simulink model "CM670A_HwAg1Meas"  (R2013b)
settings: Solver=FixedStepDiscrete  SolverMode=SingleTasking  StartTime=0.0  StopTime=22  FixedStep=0.002  RelTol=1e-3
values from neighbouring files (symbols this model uses):
  ELECGLBPRM_DEGPERREV_DEGPERREV_F32 = DataDict.Constant    [CM670A_HwAg1Meas_DataDict.m]
  ELECGLBPRM_HWAGCENTROFFS_HWDEG_F32 = DataDict.Constant    [CM670A_HwAg1Meas_DataDict.m]
  ELECGLBPRM_HWAGSATNLOWRLIM_HWDEG_F32 = DataDict.Constant    [CM670A_HwAg1Meas_DataDict.m]
  ELECGLBPRM_HWAGSATNUPPRLIM_HWDEG_F32 = DataDict.Constant    [CM670A_HwAg1Meas_DataDict.m]
  ELECGLBPRM_HWAGSCA_ULS_F32 = DataDict.Constant    [CM670A_HwAg1Meas_DataDict.m]
  ELECGLBPRM_HWAGSPURGEARRAT_ULS_F32 = DataDict.Constant    [CM670A_HwAg1Meas_DataDict.m]
  ELECGLBPRM_HWAGSPURTORINGGEARRATSNSR0_ULS_F32 = DataDict.Constant    [CM670A_HwAg1Meas_DataDict.m]
  ELECGLBPRM_HWAGSPURTORINGGEARRATSNSR1_ULS_F32 = DataDict.Constant    [CM670A_HwAg1Meas_DataDict.m]
  ELECGLBPRM_NOFLT_CNT_U08 = DataDict.Constant    [CM670A_HwAg1Meas_DataDict.m]
  ELECGLBPRM_OFFSTRIMNOTPRFMD_CNT_U08 = DataDict.Constant    [CM670A_HwAg1Meas_DataDict.m]
  ELECGLBPRM_PRTCLFLT_CNT_U08 = DataDict.Constant    [CM670A_HwAg1Meas_DataDict.m]
  ELECGLBPRM_SKIPSTEPFLT_CNT_U08 = DataDict.Constant    [CM670A_HwAg1Meas_DataDict.m]
  ELECGLBPRM_SNSRINTFLT_CNT_U08 = DataDict.Constant    [CM670A_HwAg1Meas_DataDict.m]
  ELECGLBPRM_VRNRERRFLT_CNT_U08 = DataDict.Constant    [CM670A_HwAg1Meas_DataDict.m]
  HWAG10THTOOTHTRIG_CNT_U08 = DataDict.ConfigParam    [CM670A_HwAg1Meas_DataDict.m]
  HWAG11THTOOTHTRIG_CNT_U08 = DataDict.ConfigParam    [CM670A_HwAg1Meas_DataDict.m]
  HwAg1IfFlt = DataDict.NTC    [CM670A_HwAg1Meas_DataDict.m]
  HwAg1MeasHwAg1IfFltFailStep = DataDict.Calibration    [CM670A_HwAg1Meas_DataDict.m]
  HwAg1MeasHwAg1IfFltPassStep = DataDict.Calibration    [CM670A_HwAg1Meas_DataDict.m]
  HwAg1MeasHwAg1Snsr0PrtclFltFailStep = DataDict.Calibration    [CM670A_HwAg1Meas_DataDict.m]
  HwAg1MeasHwAg1Snsr0PrtclFltPassStep = DataDict.Calibration    [CM670A_HwAg1Meas_DataDict.m]
  HwAg1MeasHwAg1Snsr1PrtclFltFailStep = DataDict.Calibration    [CM670A_HwAg1Meas_DataDict.m]
  HwAg1MeasHwAg1Snsr1PrtclFltPassStep = DataDict.Calibration    [CM670A_HwAg1Meas_DataDict.m]
  HwAg1MeasSnsr0Rev = DataDict.Calibration    [CM670A_HwAg1Meas_DataDict.m]
  HwAg1MeasSnsr1Rev = DataDict.Calibration    [CM670A_HwAg1Meas_DataDict.m]
  HwAg1MeasStep = DataDict.Calibration    [CM670A_HwAg1Meas_DataDict.m]
  HwAg1MeasVrnrErrThd = DataDict.Calibration    [CM670A_HwAg1Meas_DataDict.m]
  HwAg1MfgFlt = DataDict.NTC    [CM670A_HwAg1Meas_DataDict.m]
  HwAg1Snsr0PrtclFlt = DataDict.NTC    [CM670A_HwAg1Meas_DataDict.m]
  HwAg1Snsr1PrtclFlt = DataDict.NTC    [CM670A_HwAg1Meas_DataDict.m]
undefined symbols (not defined in the file or in its folder): NtcSts1, sigbuilder_block, SigQlfr1
libraries: simulink x30, NxtrNvM x3
(part 4 of 5)

== system CM670A_HwAg1Meas/HwAg1Meas/HwAg1MeasPer4/HwAgRead/If Action Subsystem3 ==
  Action Port : ActionPort  ActionType=else
  CopyRight2 : Subsystem  Description=|  mask(Copyright Information){none=on}
      | Copyright info block.                                               
      |                                                                     
      | Place copyright information at the top of every subsystem in design.
      mask prompts: none "No parameters"
      mask help: Place copyright information at the top of every subsystem in design.
      mask Display:
      | NxtrConf = 'Nexteer Confidential';
      | 
      | sys = bdroot; %handle for the current model ("system")
      | first = get_param(sys,'Created');
      | first = first(end-3:end);  %year is last four digits
      | 
      | last = get_param(sys,'LastModifiedDate');
      | if isempty(last)
      |     last = datestr(now,'yyyy');
      | else
      |     last = last(end-3:end);
      | end
      | 
      | if strcmp(first,last)
      |     fprintf('%s -- Copyright %s Nexteer',NxtrConf,first)
      | else
      |     fprintf('%s -- %s%s- %s Nexteer',NxtrConf,char(169),first,last)
      | end
  Data Type Conversion : DataTypeConversion  OutDataTypeStr=uint8
  SigQlfr : simulink/Sources/Enumerated Constant  OutDataTypeStr=Enum: SigQlfr1  Value=SigQlfr1.SIGQLFR_FAILD  SampleTime=inf
  Qlfr : Outport
  wires:
  SigQlfr/1 -> Data Type Conversion/1
  Data Type Conversion/1 -> Qlfr/1

== system CM670A_HwAg1Meas/HwAg1Meas/HwAg1MeasPer5/If Action Subsystem/CopyRight2 ==

== system CM670A_HwAg1Meas/HwAg1Meas/HwAg1MeasPer5/If Action Subsystem1/CopyRight2 ==

== system CM670A_HwAg1Meas/HwAg1Meas/HwAg1MeasPer5/SetNtcSts/CopyRight2 ==

== system CM670A_HwAg1Meas/HwAg1Meas/HwAg1MeasPer2/Snsr0Read/DebStepSelection/CopyRight2 ==

== system CM670A_HwAg1Meas/HwAg1Meas/HwAg1MeasPer2/Snsr0Read/Do nothing/CopyRight2 ==

== system CM670A_HwAg1Meas/HwAg1Meas/HwAg1MeasPer2/Snsr0Read/RawHwAgRead/CopyRight2 ==

== system CM670A_HwAg1Meas/HwAg1Meas/HwAg1MeasPer2/Snsr0Read/RawHwAgRead/NewMsg ==
  note: Information Only:
      |
      | - Protocol Fault Evaluation
  Snsr0CS : Inport
  Snsr0FCCN : Inport  Port=2
  Snsr0Id : Inport  Port=3
  Snsr0Data : Inport  Port=4
  Action Port : ActionPort  ActionType=then
  Bus Creator : BusCreator  Inputs=3
  Bus Selector : BusSelector  OutputSignals=RawHwAg,TestOk,ParamByte
  Bus Selector1 : BusSelector  OutputSignals=RawHwAg,TestOk,ParamByte
  CopyRight2 : Subsystem  Description=|  mask(Copyright Information){none=on}
      | Copyright info block.                                               
      |                                                                     
      | Place copyright information at the top of every subsystem in design.
      mask prompts: none "No parameters"
      mask help: Place copyright information at the top of every subsystem in design.
      mask Display:
      | NxtrConf = 'Nexteer Confidential';
      | 
      | sys = bdroot; %handle for the current model ("system")
      | first = get_param(sys,'Created');
      | first = first(end-3:end);  %year is last four digits
      | 
      | last = get_param(sys,'LastModifiedDate');
      | if isempty(last)
      |     last = datestr(now,'yyyy');
      | else
      |     last = last(end-3:end);
      | end
      | 
      | if strcmp(first,last)
      |     fprintf('%s -- Copyright %s Nexteer',NxtrConf,first)
      | else
      |     fprintf('%s -- %s%s- %s Nexteer',NxtrConf,char(169),first,last)
      | end
  If : If  RequirementInfo={} %GIDa_5864e763_b026_443d_97f3_5968bd211996  IfExpression=u1 == 0
  Merge : Merge
  Merge1 : Merge
  Merge2 : Merge
  NoStsFlt : Subsystem  RequirementInfo={} %GIDa_3d7633e9_7103_42ab_9daf_68a78569a74b  TreatAsAtomicUnit=on
  STSFLT : Subsystem  RequirementInfo={'linktype_rmi_doors' '0000cf44 (/ESG Group/FDD Module Requirements/EA4 Specific/CM670A_HwAg1Meas)' '#CM670A_40' 'true' 'REQ: CM670A_40' '' ; 'linktype_rmi_doors' '0000cf44 (/ESG Group/FDD Module Requirements/EA4 Specific/CM670A_HwAg1Meas)' '#CM670A_41' 'true' 'REQ: CM670A_41' '' ; 'linktype_rmi_doors' '0000cf44 (/ESG Group/FDD Module Requirements/EA4 Specific/CM670A_HwAg1Meas)' '#CM670A_42' 'true' 'REQ: CM670A_42' '' ; 'linktype_rmi_doors' '0000cf44 (/ESG Group/FDD Module Requirements/EA4 Specific/CM670A_HwAg1Meas)' '#CM670A_43' 'true' 'REQ: CM670A_43' '' ; 'linktype_rmi_doors' '0000cf44 (/ESG Group/FDD Module Requirements/EA4 Specific/CM670A_HwAg1Meas)' '#CM670A_44' 'true' 'REQ: CM670A_44' '' ; 'linktype_rmi_doors' '0000cf44 (/ESG Group/FDD Module Requirements/EA4 Specific/CM670A_HwAg1Meas)' '#CM670A_45' 'true' 'REQ: CM670A_45' '' ; 'linktype_rmi_doors' '0000cf44 (/ESG Group/FDD Module Requirements/EA4 Specific/CM670A_HwAg1Meas)' '#CM670A_46' 'true' 'REQ: CM670A_46' '' ; 'linktype_rmi_doors' '0000cf44 (/ESG Group/FDD Module Requirements/EA4 Specific/CM670A_HwAg1Meas)' '#CM670A_55' 'true' 'REQ: CM670A_55' '' } %GIDa_baa7679c_fb57_46f2_9762_1b097a58bedf  TreatAsAtomicUnit=on
      mask Display: disp('STSFLT')
  Out1 : Outport
  wires:
  If/1 -> NoStsFlt/Action  "NoFault"
  If/2 -> STSFLT/Action  "Fault"
  Merge/1 -> Bus Creator/2  "TestOk"
  Merge1/1 -> Bus Creator/3  "ParamByte"
  Merge2/1 -> Bus Creator/1  "RawHwAg"
  NoStsFlt/1(Out1) -> Bus Selector/1
  STSFLT/1(Out1) -> Bus Selector1/1
  Bus Selector1/1 -> Merge2/1  "<RawHwAg>"
  Bus Selector/1 -> Merge2/2  "<RawHwAg>"
  Bus Selector1/2 -> Merge/1  "<TestOk>"
  Bus Selector1/3 -> Merge1/1  "<ParamByte>"
  Bus Selector/2 -> Merge/2  "<TestOk>"
  Bus Selector/3 -> Merge1/2  "<ParamByte>"
  Bus Creator/1 -> Out1/1
  Snsr0CS/1 -> If/1
  Snsr0FCCN/1 -> NoStsFlt/1(Snsr0FCCN)
  Snsr0Data/1 -> NoStsFlt/3(Snsr0Data)
  Snsr0Id/1 -> NoStsFlt/2(Snsr0Id)

== system CM670A_HwAg1Meas/HwAg1Meas/HwAg1MeasPer2/Snsr0Read/RawHwAgRead/NoNewMsg ==
  Action Port : ActionPort  ActionType=else
  Add : Sum
  Bus Creator : BusCreator  Inputs=3
  Constant : Constant  OutDataTypeStr=uint8
  CopyRight2 : Subsystem  Description=|  mask(Copyright Information){none=on}
      | Copyright info block.                                               
      |                                                                     
      | Place copyright information at the top of every subsystem in design.
      mask prompts: none "No parameters"
      mask help: Place copyright information at the top of every subsystem in design.
      mask Display:
      | NxtrConf = 'Nexteer Confidential';
      | 
      | sys = bdroot; %handle for the current model ("system")
      | first = get_param(sys,'Created');
      | first = first(end-3:end);  %year is last four digits
      | 
      | last = get_param(sys,'LastModifiedDate');
      | if isempty(last)
      |     last = datestr(now,'yyyy');
      | else
      |     last = last(end-3:end);
      | end
      | 
      | if strcmp(first,last)
      |     fprintf('%s -- Copyright %s Nexteer',NxtrConf,first)
      | else
      |     fprintf('%s -- %s%s- %s Nexteer',NxtrConf,char(169),first,last)
      | end
  Data Store Read : DataStoreRead  DataStoreName=HwAg1Snsr0NoMsgErrCntr
  Data Store Write : DataStoreWrite  DataStoreName=HwAg1Snsr0NoMsgErrCntr
  Data Type Conversion : DataTypeConversion  OutDataTypeStr=uint8
  HwAg : Constant  Value=0  OutDataTypeStr=uint16
  NtcSts : simulink/Sources/Enumerated Constant  OutDataTypeStr=Enum: NtcSts1  Value=NtcSts1.NTCSTS_PREFAILD  SampleTime=inf
  PRTCL_FAULT : Constant  Value=ELECGLBPRM_PRTCLFLT_CNT_U08  OutDataTypeStr=uint8
  Signal Conversion : SignalConversion
  Out1 : Outport
  wires:
  PRTCL_FAULT/1 -> Bus Creator/3  "ParamByte"
  NtcSts/1 -> Data Type Conversion/1
  HwAg/1 -> Bus Creator/1  "RawHwAg"
  Bus Creator/1 -> Signal Conversion/1
  Signal Conversion/1 -> Out1/1
  Data Type Conversion/1 -> Bus Creator/2  "TestOk"
  Data Store Read/1 -> Add/1
  Constant/1 -> Add/2
  Add/1 -> Data Store Write/1

== system CM670A_HwAg1Meas/HwAg1Meas/HwAg1MeasPer2/Snsr0Read/Read the Flag/CopyRight2 ==

== system CM670A_HwAg1Meas/HwAg1Meas/HwAg1MeasPer2/Snsr0Read/SetNtcSts/CopyRight2 ==

== system CM670A_HwAg1Meas/HwAg1Meas/HwAg1MeasPer3/Snsr1Read/DebStepSelection/CopyRight2 ==

== system CM670A_HwAg1Meas/HwAg1Meas/HwAg1MeasPer3/Snsr1Read/Do nothing/CopyRight2 ==

== system CM670A_HwAg1Meas/HwAg1Meas/HwAg1MeasPer3/Snsr1Read/Do nothing1/CopyRight2 ==

== system CM670A_HwAg1Meas/HwAg1Meas/HwAg1MeasPer3/Snsr1Read/RawHwAgRead/CopyRight2 ==

== system CM670A_HwAg1Meas/HwAg1Meas/HwAg1MeasPer3/Snsr1Read/RawHwAgRead/NewMsg ==
  note: Information Only:
      |
      | - Protocol Fault Evaluation
  Snsr1CS : Inport
  Snsr1FCCN : Inport  Port=2
  Snsr1Id : Inport  Port=3
  Snsr1Data : Inport  Port=4
  Action Port : ActionPort  ActionType=then
  Bus Creator : BusCreator  Inputs=3
  Bus Selector : BusSelector  OutputSignals=RawHwAg,TestOk,ParamByte
  Bus Selector1 : BusSelector  OutputSignals=RawHwAg,TestOk,ParamByte
  CopyRight2 : Subsystem  Description=|  mask(Copyright Information){none=on}
      | Copyright info block.                                               
      |                                                                     
      | Place copyright information at the top of every subsystem in design.
      mask prompts: none "No parameters"
      mask help: Place copyright information at the top of every subsystem in design.
      mask Display:
      | NxtrConf = 'Nexteer Confidential';
      | 
      | sys = bdroot; %handle for the current model ("system")
      | first = get_param(sys,'Created');
      | first = first(end-3:end);  %year is last four digits
      | 
      | last = get_param(sys,'LastModifiedDate');
      | if isempty(last)
      |     last = datestr(now,'yyyy');
      | else
      |     last = last(end-3:end);
      | end
      | 
      | if strcmp(first,last)
      |     fprintf('%s -- Copyright %s Nexteer',NxtrConf,first)
      | else
      |     fprintf('%s -- %s%s- %s Nexteer',NxtrConf,char(169),first,last)
      | end
  If : If  RequirementInfo={} %GIDa_181674f6_4b7d_42d7_8f8c_71fbeb7e558d  IfExpression=u1 == 0
  Merge : Merge
  Merge1 : Merge
  Merge2 : Merge
  NoStsFlt : Subsystem  RequirementInfo={} %GIDa_72d33f52_5760_4aac_8869_08591bcc9dca  TreatAsAtomicUnit=on
  STSFLT : Subsystem  RequirementInfo={'linktype_rmi_doors' '0000cf44 (/ESG Group/FDD Module Requirements/EA4 Specific/CM670A_HwAg1Meas)' '#CM670A_62' 'true' 'REQ: CM670A_62' '' ; 'linktype_rmi_doors' '0000cf44 (/ESG Group/FDD Module Requirements/EA4 Specific/CM670A_HwAg1Meas)' '#CM670A_63' 'true' 'REQ: CM670A_63' '' ; 'linktype_rmi_doors' '0000cf44 (/ESG Group/FDD Module Requirements/EA4 Specific/CM670A_HwAg1Meas)' '#CM670A_64' 'true' 'REQ: CM670A_64' '' ; 'linktype_rmi_doors' '0000cf44 (/ESG Group/FDD Module Requirements/EA4 Specific/CM670A_HwAg1Meas)' '#CM670A_65' 'true' 'REQ: CM670A_65' '' ; 'linktype_rmi_doors' '0000cf44 (/ESG Group/FDD Module Requirements/EA4 Specific/CM670A_HwAg1Meas)' '#CM670A_66' 'true' 'REQ: CM670A_66' '' ; 'linktype_rmi_doors' '0000cf44 (/ESG Group/FDD Module Requirements/EA4 Specific/CM670A_HwAg1Meas)' '#CM670A_67' 'true' 'REQ: CM670A_67' '' ; 'linktype_rmi_doors' '0000cf44 (/ESG Group/FDD Module Requirements/EA4 Specific/CM670A_HwAg1Meas)' '#CM670A_68' 'true' 'REQ: CM670A_68' '' ; 'linktype_rmi_doors' '0000cf44 (/ESG Group/FDD Module Requirements/EA4 Specific/CM670A_HwAg1Meas)' '#CM670A_69' 'true' 'REQ: CM670A_69' '' } %GIDa_cab96659_2f05_48ba_9310_e516fce1dae6  TreatAsAtomicUnit=on
      mask Display: disp('STSFLT')
  Out1 : Outport
  wires:
  If/1 -> NoStsFlt/Action  "NoFault"
  If/2 -> STSFLT/Action  "Fault"
  Merge/1 -> Bus Creator/2  "TestOk"
  Merge1/1 -> Bus Creator/3  "ParamByte"
  Merge2/1 -> Bus Creator/1  "RawHwAg"
  NoStsFlt/1(Out1) -> Bus Selector/1
  STSFLT/1(Out1) -> Bus Selector1/1
  Bus Selector1/1 -> Merge2/1  "<RawHwAg>"
  Bus Selector/1 -> Merge2/2  "<RawHwAg>"
  Bus Selector1/2 -> Merge/1  "<TestOk>"
  Bus Selector1/3 -> Merge1/1  "<ParamByte>"
  Bus Selector/2 -> Merge/2  "<TestOk>"
  Bus Selector/3 -> Merge1/2  "<ParamByte>"
  Bus Creator/1 -> Out1/1
  Snsr1CS/1 -> If/1
  Snsr1FCCN/1 -> NoStsFlt/1(Snsr1FCCN)
  Snsr1Data/1 -> NoStsFlt/3(Snsr1Data)
  Snsr1Id/1 -> NoStsFlt/2(Snsr1Id)

== stateflow chart CM670A_HwAg1Meas/HwAg1Meas/HwAg1MeasPer4/HwAgRead/HwAg1Final/ModRoll ==
  settings: stateMachineType=MEALY_MACHINE
  note: Nexteer Automotive Confidential
  (default) -> (junction 89)
  (junction 89) -> (junction 93) [order 2] : [ RawVal>900 ]
      | {OutVal = RawVal-1800;}
  (junction 89) -> (junction 93) [order 3] : {OutVal = RawVal;}
  (junction 89) -> (junction 93) [order 1] : [RawVal<-900 ]
      | {OutVal = RawVal+1800;}
  data: OutVal output single; RawVal input single

== system CM670A_HwAg1Meas/HwAg1Meas/HwAg1MeasPer3/Snsr1Read/RawHwAgRead/NoNewMsg ==
  Action Port : ActionPort  ActionType=else
  Add : Sum
  Bus Creator : BusCreator  Inputs=3
  Constant : Constant  OutDataTypeStr=uint8
  CopyRight2 : Subsystem  Description=|  mask(Copyright Information){none=on}
      | Copyright info block.                                               
      |                                                                     
      | Place copyright information at the top of every subsystem in design.
      mask prompts: none "No parameters"
      mask help: Place copyright information at the top of every subsystem in design.
      mask Display:
      | NxtrConf = 'Nexteer Confidential';
      | 
      | sys = bdroot; %handle for the current model ("system")
      | first = get_param(sys,'Created');
      | first = first(end-3:end);  %year is last four digits
      | 
      | last = get_param(sys,'LastModifiedDate');
      | if isempty(last)
      |     last = datestr(now,'yyyy');
      | else
      |     last = last(end-3:end);
      | end
      | 
      | if strcmp(first,last)
      |     fprintf('%s -- Copyright %s Nexteer',NxtrConf,first)
      | else
      |     fprintf('%s -- %s%s- %s Nexteer',NxtrConf,char(169),first,last)
      | end
  Data Store Read : DataStoreRead  DataStoreName=HwAg1Snsr1NoMsgErrCntr
  Data Store Write : DataStoreWrite  DataStoreName=HwAg1Snsr1NoMsgErrCntr
  Data Type Conversion : DataTypeConversion  OutDataTypeStr=uint8
  HwAg : Constant  Value=0  OutDataTypeStr=uint16
  NtcSts : simulink/Sources/Enumerated Constant  OutDataTypeStr=Enum: NtcSts1  Value=NtcSts1.NTCSTS_PREFAILD  SampleTime=inf
  PRTCL_FAULT : Constant  Value=ELECGLBPRM_PRTCLFLT_CNT_U08  OutDataTypeStr=uint8
  Signal Conversion : SignalConversion
  Out1 : Outport
  wires:
  PRTCL_FAULT/1 -> Bus Creator/3  "ParamByte"
  NtcSts/1 -> Data Type Conversion/1
  HwAg/1 -> Bus Creator/1  "RawHwAg"
  Bus Creator/1 -> Signal Conversion/1
  Signal Conversion/1 -> Out1/1
  Data Type Conversion/1 -> Bus Creator/2  "TestOk"
  Data Store Read/1 -> Add/1
  Constant/1 -> Add/2
  Add/1 -> Data Store Write/1

== system CM670A_HwAg1Meas/HwAg1Meas/HwAg1MeasPer3/Snsr1Read/Read the Flag/CopyRight2 ==

== system CM670A_HwAg1Meas/HwAg1Meas/HwAg1MeasPer3/Snsr1Read/SetNtcSts/CopyRight2 ==

== system CM670A_HwAg1Meas/HwAg1Meas/HwAg1MeasPer3/Snsr1Read/SyncPulse/CopyRight2 ==

== system CM670A_HwAg1Meas/HwAg1Meas/HwAg1MeasPer3/Snsr1Read/SyncPulse/GetRefTmr1MicroSec32bit ==
  CopyRight2 : Subsystem  Description=|  mask(Copyright Information){none=on}
      | Copyright info block.                                               
      |                                                                     
      | Place copyright information at the top of every subsystem in design.
      mask prompts: none "No parameters"
      mask help: Place copyright information at the top of every subsystem in design.
      mask Display:
      | NxtrConf = 'Nexteer Confidential';
      | 
      | sys = bdroot; %handle for the current model ("system")
      | first = get_param(sys,'Created');
      | first = first(end-3:end);  %year is last four digits
      | 
      | last = get_param(sys,'LastModifiedDate');
      | if isempty(last)
      |     last = datestr(now,'yyyy');
      | else
      |     last = last(end-3:end);
      | end
      | 
      | if strcmp(first,last)
      |     fprintf('%s -- Copyright %s Nexteer',NxtrConf,first)
      | else
      |     fprintf('%s -- %s%s- %s Nexteer',NxtrConf,char(169),first,last)
      | end
  Ground : Ground
  RefTmr : Outport
  wires:
  Ground/1 -> RefTmr/1

== system CM670A_HwAg1Meas/HwAg1Meas/HwAg1MeasPer3/Snsr1Read/SyncPulse/GetTiSpan1MicroSec32bit ==
  RefTmr : Inport
  CopyRight2 : Subsystem  Description=|  mask(Copyright Information){none=on}
      | Copyright info block.                                               
      |                                                                     
      | Place copyright information at the top of every subsystem in design.
      mask prompts: none "No parameters"
      mask help: Place copyright information at the top of every subsystem in design.
      mask Display:
      | NxtrConf = 'Nexteer Confidential';
      | 
      | sys = bdroot; %handle for the current model ("system")
      | first = get_param(sys,'Created');
      | first = first(end-3:end);  %year is last four digits
      | 
      | last = get_param(sys,'LastModifiedDate');
      | if isempty(last)
      |     last = datestr(now,'yyyy');
      | else
      |     last = last(end-3:end);
      | end
      | 
      | if strcmp(first,last)
      |     fprintf('%s -- Copyright %s Nexteer',NxtrConf,first)
      | else
      |     fprintf('%s -- %s%s- %s Nexteer',NxtrConf,char(169),first,last)
      | end
  Ground : Ground
  Terminator : Terminator
  TiSpan : Outport
  wires:
  RefTmr/1 -> Terminator/1
  Ground/1 -> TiSpan/1

== system CM670A_HwAg1Meas/HwAg1Meas/HwAg1MeasPer4/HwAgRead/GetNtcQlfr/CopyRight2 ==

== system CM670A_HwAg1Meas/HwAg1Meas/HwAg1MeasPer4/HwAgRead/GetNtcQlfr1/CopyRight2 ==

== system CM670A_HwAg1Meas/HwAg1Meas/HwAg1MeasPer4/HwAgRead/GetNtcQlfr2/CopyRight2 ==

== system CM670A_HwAg1Meas/HwAg1Meas/HwAg1MeasPer4/HwAgRead/GetNtcQlfr3/CopyRight2 ==

== system CM670A_HwAg1Meas/HwAg1Meas/HwAg1MeasPer4/HwAgRead/HwAg1Final/CopyRight2 ==

== system CM670A_HwAg1Meas/HwAg1Meas/HwAg1MeasPer4/HwAgRead/If Action Subsystem/AdjStepCalc ==
  HwAg1Snsr0Rel : Inport
  HwAg1Sns1Rel : Inport  Port=2
  CopyRight2 : Subsystem  Description=|  mask(Copyright Information){none=on}
      | Copyright info block.                                               
      |                                                                     
      | Place copyright information at the top of every subsystem in design.
      mask prompts: none "No parameters"
      mask help: Place copyright information at the top of every subsystem in design.
      mask Display:
      | NxtrConf = 'Nexteer Confidential';
      | 
      | sys = bdroot; %handle for the current model ("system")
      | first = get_param(sys,'Created');
      | first = first(end-3:end);  %year is last four digits
      | 
      | last = get_param(sys,'LastModifiedDate');
      | if isempty(last)
      |     last = datestr(now,'yyyy');
      | else
      |     last = last(end-3:end);
      | end
      | 
      | if strcmp(first,last)
      |     fprintf('%s -- Copyright %s Nexteer',NxtrConf,first)
      | else
      |     fprintf('%s -- %s%s- %s Nexteer',NxtrConf,char(169),first,last)
      | end
  Diagc : Subsystem
  InitStep : Subsystem
      settings: AttributesFormatString=%<Description>
  Intpn : Subsystem
  HwAg1 : Outport  OutDataTypeStr=single
  TestOk : Outport  Port=2  OutDataTypeStr=uint8
  ParamByte : Outport  Port=3
  wires:
  HwAg1Sns1Rel/1 -> Diagc/2(HwAg1Snsr1Rel), Intpn/2(HwAg1Snsr1Rel)
  HwAg1Snsr0Rel/1 -> Intpn/1(HwAg1Snsr0Rel), Diagc/1(HwAg1Snsr0Rel)
  Diagc/1(HwAg1) -> HwAg1/1
  Diagc/2(TestOk) -> TestOk/1
  Diagc/3(ParamByte) -> ParamByte/1
  Intpn/1(HwAg1Snsr0Rev) -> Diagc/3(HwAg1Snsr0Rev)
  Intpn/2(HwAg1Snsr1Rev) -> Diagc/4(HwAg1Snsr1Rev)
  Intpn/3(HwAg1StepSeqNr) -> InitStep/1(HwAg1StepSeqNr_In)
  InitStep/1(HwAg1StepSeqNr_Out) -> Diagc/5(HwAg1StepSeqNr)

== system CM670A_HwAg1Meas/HwAg1Meas/HwAg1MeasPer4/HwAgRead/If Action Subsystem/CopyRight2 ==

== system CM670A_HwAg1Meas/HwAg1Meas/HwAg1MeasPer4/HwAgRead/If Action Subsystem/DebStepSelection ==
  TestOk : Inport
  CopyRight2 : Subsystem  Description=|  mask(Copyright Information){none=on}
      | Copyright info block.                                               
      |                                                                     
      | Place copyright information at the top of every subsystem in design.
      mask prompts: none "No parameters"
      mask help: Place copyright information at the top of every subsystem in design.
      mask Display:
      | NxtrConf = 'Nexteer Confidential';
      | 
      | sys = bdroot; %handle for the current model ("system")
      | first = get_param(sys,'Created');
      | first = first(end-3:end);  %year is last four digits
      | 
      | last = get_param(sys,'LastModifiedDate');
      | if isempty(last)
      |     last = datestr(now,'yyyy');
      | else
      |     last = last(end-3:end);
      | end
      | 
      | if strcmp(first,last)
      |     fprintf('%s -- Copyright %s Nexteer',NxtrConf,first)
      | else
      |     fprintf('%s -- %s%s- %s Nexteer',NxtrConf,char(169),first,last)
      | end
  NTCFailStepCal : Constant  Value=HwAg1MeasHwAg1IfFltFailStep
  NTCPassStepCal : Constant  Value=HwAg1MeasHwAg1IfFltPassStep
  Switch : Switch  Criteria=u2 > Threshold  Threshold=2
  DebStep : Outport  OutDataTypeStr=uint16
  wires:
  NTCFailStepCal/1 -> Switch/1
  Switch/1 -> DebStep/1
  NTCPassStepCal/1 -> Switch/3
  TestOk/1 -> Switch/2

== system CM670A_HwAg1Meas/HwAg1Meas/HwAg1MeasPer4/HwAgRead/If Action Subsystem/HwAg1Snsr0RelCalc ==
  RawHwAg1Snsr0 : Inport
  CopyRight2 : Subsystem  Description=|  mask(Copyright Information){none=on}
      | Copyright info block.                                               
      |                                                                     
      | Place copyright information at the top of every subsystem in design.
      mask prompts: none "No parameters"
      mask help: Place copyright information at the top of every subsystem in design.
      mask Display:
      | NxtrConf = 'Nexteer Confidential';
      | 
      | sys = bdroot; %handle for the current model ("system")
      | first = get_param(sys,'Created');
      | first = first(end-3:end);  %year is last four digits
      | 
      | last = get_param(sys,'LastModifiedDate');
      | if isempty(last)
      |     last = datestr(now,'yyyy');
      | else
      |     last = last(end-3:end);
      | end
      | 
      | if strcmp(first,last)
      |     fprintf('%s -- Copyright %s Nexteer',NxtrConf,first)
      | else
      |     fprintf('%s -- %s%s- %s Nexteer',NxtrConf,char(169),first,last)
      | end
  Data Type Conversion1 : DataTypeConversion  OutDataTypeStr=single
  HwAgSca : Constant  Value=ELECGLBPRM_HWAGSCA_ULS_F32  OutDataTypeStr=single
  PIM : DataStoreWrite  RequirementInfo={} %GIDa_13b8254a_99fe_44d8_b113_6d22cedea98d  DataStoreName=dHwAg1MeasSnsr0Rel
  Product : Product
  HwAg1Snsr0Rel : Outport  OutDataTypeStr=single
  wires:
  Data Type Conversion1/1 -> Product/1
  RawHwAg1Snsr0/1 -> Data Type Conversion1/1
  HwAgSca/1 -> Product/2
  Product/1 -> PIM/1, HwAg1Snsr0Rel/1

== system CM670A_HwAg1Meas/HwAg1Meas/HwAg1MeasPer4/HwAgRead/If Action Subsystem/HwAg1Snsr1RelCalc ==
  RawHwAg1Snsr1 : Inport
  CopyRight2 : Subsystem  Description=|  mask(Copyright Information){none=on}
      | Copyright info block.                                               
      |                                                                     
      | Place copyright information at the top of every subsystem in design.
      mask prompts: none "No parameters"
      mask help: Place copyright information at the top of every subsystem in design.
      mask Display:
      | NxtrConf = 'Nexteer Confidential';
      | 
      | sys = bdroot; %handle for the current model ("system")
      | first = get_param(sys,'Created');
      | first = first(end-3:end);  %year is last four digits
      | 
      | last = get_param(sys,'LastModifiedDate');
      | if isempty(last)
      |     last = datestr(now,'yyyy');
      | else
      |     last = last(end-3:end);
      | end
      | 
      | if strcmp(first,last)
      |     fprintf('%s -- Copyright %s Nexteer',NxtrConf,first)
      | else
      |     fprintf('%s -- %s%s- %s Nexteer',NxtrConf,char(169),first,last)
      | end
  Data Type Conversion1 : DataTypeConversion  OutDataTypeStr=single
  HwAgSca : Constant  Value=ELECGLBPRM_HWAGSCA_ULS_F32  OutDataTypeStr=single
  PIM : DataStoreWrite  RequirementInfo={} %GIDa_b01eea6e_937c_45e5_83b1_7742cf1179bc  DataStoreName=dHwAg1MeasSnsr1Rel
  Product : Product
  HwAg1Snsr1Rel : Outport  OutDataTypeStr=single
  wires:
  Data Type Conversion1/1 -> Product/1
  RawHwAg1Snsr1/1 -> Data Type Conversion1/1
  HwAgSca/1 -> Product/2
  Product/1 -> PIM/1, HwAg1Snsr1Rel/1

== system CM670A_HwAg1Meas/HwAg1Meas/HwAg1MeasPer4/HwAgRead/If Action Subsystem/SetNtcSts ==
  note: Note:
      |
      | - "ISO Fault Debounce Design" Simulink block intent to use here for Simulation purpose only. Do not Code this block
  NtcNr : Inport
  NtcStInfo : Inport  Port=2
  NtcSts : Inport  Port=3
  DebStep : Inport  Port=4
  CopyRight2 : Subsystem  Description=|  mask(Copyright Information){none=on}
      | Copyright info block.                                               
      |                                                                     
      | Place copyright information at the top of every subsystem in design.
      mask prompts: none "No parameters"
      mask help: Place copyright information at the top of every subsystem in design.
      mask Display:
      | NxtrConf = 'Nexteer Confidential';
      | 
      | sys = bdroot; %handle for the current model ("system")
      | first = get_param(sys,'Created');
      | first = first(end-3:end);  %year is last four digits
      | 
      | last = get_param(sys,'LastModifiedDate');
      | if isempty(last)
      |     last = datestr(now,'yyyy');
      | else
      |     last = last(end-3:end);
      | end
      | 
      | if strcmp(first,last)
      |     fprintf('%s -- Copyright %s Nexteer',NxtrConf,first)
      | else
      |     fprintf('%s -- %s%s- %s Nexteer',NxtrConf,char(169),first,last)
      | end
  Data Store Write : DataStoreWrite  DataStoreName=Ntc0x098Qlfr
  Ground : Ground
  ISO Fault Debounce Design : Stateflow chart  TreatAsAtomicUnit=on
      settings: AttributesFormatString=|
      | Simulation Purpose Only.
      | Do Not Code this block
      | Diagnostic Manager Owns this requirement
  Scope1 : Scope  NumInputPorts=3
      settings: YMin=-5~-5~-5  YMax=5~5~5  SaveName=ScopeData5
  Terminator : Terminator
  Terminator1 : Terminator
  wires:
  Ground/1 -> ISO Fault Debounce Design/3(SvcClr)
  ISO Fault Debounce Design/1(Qualifier) -> Data Store Write/1, Scope1/3
  DebStep/1 -> Scope1/2, ISO Fault Debounce Design/2(DebStep)
  NtcSts/1 -> Scope1/1, ISO Fault Debounce Design/1(NtcSts)
  NtcNr/1 -> Terminator/1
  NtcStInfo/1 -> Terminator1/1

== system CM670A_HwAg1Meas/HwAg1Meas/HwAg1MeasPer4/HwAgRead/If Action Subsystem1/CopyRight2 ==

== system CM670A_HwAg1Meas/HwAg1Meas/HwAg1MeasPer4/HwAgRead/If Action Subsystem2/CopyRight2 ==

== system CM670A_HwAg1Meas/HwAg1Meas/HwAg1MeasPer4/HwAgRead/If Action Subsystem3/CopyRight2 ==

== system CM670A_HwAg1Meas/HwAg1Meas/HwAg1MeasPer2/Snsr0Read/RawHwAgRead/NewMsg/CopyRight2 ==

== system CM670A_HwAg1Meas/HwAg1Meas/HwAg1MeasPer2/Snsr0Read/RawHwAgRead/NewMsg/NoStsFlt ==
  note: Information Only:
      |
      | - Sensor Internal Fault (Status and Communication Nibble)
  Snsr0FCCN : Inport
  Snsr0Id : Inport  Port=2
  Snsr0Data : Inport  Port=3
  Action Port : ActionPort  ActionType=then
  Bus Creator : BusCreator  Inputs=3
  Bus Selector : BusSelector  OutputSignals=RawHwAg,TestOk,ParamByte
  Bus Selector1 : BusSelector  OutputSignals=RawHwAg,TestOk,ParamByte
  CommFlt : Subsystem  RequirementInfo={'linktype_rmi_doors' '0000cf44 (/ESG Group/FDD Module Requirements/EA4 Specific/CM670A_HwAg1Meas)' '#CM670A_48' 'true' 'REQ: CM670A_48' '' ; 'linktype_rmi_doors' '0000cf44 (/ESG Group/FDD Module Requirements/EA4 Specific/CM670A_HwAg1Meas)' '#CM670A_28' 'true' 'REQ: CM670A_28' '' } %GIDa_6dd8b926_62f2_466c_baff_5d347e0a7b20  TreatAsAtomicUnit=on
      mask Display: disp('CommFlt')
  CopyRight2 : Subsystem  Description=|  mask(Copyright Information){none=on}
      | Copyright info block.                                               
      |                                                                     
      | Place copyright information at the top of every subsystem in design.
      mask prompts: none "No parameters"
      mask help: Place copyright information at the top of every subsystem in design.
      mask Display:
      | NxtrConf = 'Nexteer Confidential';
      | 
      | sys = bdroot; %handle for the current model ("system")
      | first = get_param(sys,'Created');
      | first = first(end-3:end);  %year is last four digits
      | 
      | last = get_param(sys,'LastModifiedDate');
      | if isempty(last)
      |     last = datestr(now,'yyyy');
      | else
      |     last = last(end-3:end);
      | end
      | 
      | if strcmp(first,last)
      |     fprintf('%s -- Copyright %s Nexteer',NxtrConf,first)
      | else
      |     fprintf('%s -- %s%s- %s Nexteer',NxtrConf,char(169),first,last)
      | end
  If : If  IfExpression=u1 == 0
  Merge : Merge
  Merge1 : Merge
  Merge2 : Merge
  TestPass : Subsystem  TreatAsAtomicUnit=on
  Out1 : Outport
  wires:
  Snsr0FCCN/1 -> If/1
  If/1 -> TestPass/Action
  If/2 -> CommFlt/Action
  Merge/1 -> Bus Creator/2  "TestOk"
  Merge1/1 -> Bus Creator/3  "ParamByte"
  Merge2/1 -> Bus Creator/1  "RawHwAg"
  TestPass/1(Out1) -> Bus Selector/1
  CommFlt/1(Out2) -> Bus Selector1/1
  Bus Selector1/1 -> Merge2/1  "<RawHwAg>"
  Bus Selector/1 -> Merge2/2  "<RawHwAg>"
  Bus Selector1/2 -> Merge/1  "<TestOk>"
  Bus Selector1/3 -> Merge1/1  "<ParamByte>"
  Bus Selector/2 -> Merge/2  "<TestOk>"
  Bus Selector/3 -> Merge1/2  "<ParamByte>"
  Bus Creator/1 -> Out1/1
  Snsr0Data/1 -> TestPass/2(Snsr0Data)
  Snsr0Id/1 -> TestPass/1(Snsr0Id)

== system CM670A_HwAg1Meas/HwAg1Meas/HwAg1MeasPer2/Snsr0Read/RawHwAgRead/NewMsg/STSFLT ==
  Action Port : ActionPort  ActionType=else
  Add : Sum
  Bus Creator : BusCreator  Inputs=3
  Constant : Constant  OutDataTypeStr=uint8
  CopyRight2 : Subsystem  Description=|  mask(Copyright Information){none=on}
      | Copyright info block.                                               
      |                                                                     
      | Place copyright information at the top of every subsystem in design.
      mask prompts: none "No parameters"
      mask help: Place copyright information at the top of every subsystem in design.
      mask Display:
      | NxtrConf = 'Nexteer Confidential';
      | 
      | sys = bdroot; %handle for the current model ("system")
      | first = get_param(sys,'Created');
      | first = first(end-3:end);  %year is last four digits
      | 
      | last = get_param(sys,'LastModifiedDate');
      | if isempty(last)
      |     last = datestr(now,'yyyy');
      | else
      |     last = last(end-3:end);
      | end
      | 
      | if strcmp(first,last)
      |     fprintf('%s -- Copyright %s Nexteer',NxtrConf,first)
      | else
      |     fprintf('%s -- %s%s- %s Nexteer',NxtrConf,char(169),first,last)
      | end
  Data Store Read : DataStoreRead  DataStoreName=HwAg1Snsr0ComStsErrCntr
  Data Store Write : DataStoreWrite  DataStoreName=HwAg1Snsr0ComStsErrCntr
  Data Type Conversion : DataTypeConversion  OutDataTypeStr=uint8
  HwAg : Constant  Value=0  OutDataTypeStr=uint16
  NtcSts : simulink/Sources/Enumerated Constant  OutDataTypeStr=Enum: NtcSts1  Value=NtcSts1.NTCSTS_PREFAILD  SampleTime=inf
  PRTCL_FAULT : Constant  Value=ELECGLBPRM_PRTCLFLT_CNT_U08  OutDataTypeStr=uint8
  Signal Conversion : SignalConversion
  Out1 : Outport
  wires:
  PRTCL_FAULT/1 -> Bus Creator/3  "ParamByte"
  NtcSts/1 -> Data Type Conversion/1
  HwAg/1 -> Bus Creator/1  "RawHwAg"
  Bus Creator/1 -> Signal Conversion/1
  Signal Conversion/1 -> Out1/1
  Data Type Conversion/1 -> Bus Creator/2  "TestOk"
  Data Store Read/1 -> Add/1
  Constant/1 -> Add/2
  Add/1 -> Data Store Write/1

== system CM670A_HwAg1Meas/HwAg1Meas/HwAg1MeasPer2/Snsr0Read/RawHwAgRead/NoNewMsg/CopyRight2 ==

== system CM670A_HwAg1Meas/HwAg1Meas/HwAg1MeasPer3/Snsr1Read/RawHwAgRead/NewMsg/CopyRight2 ==

== system CM670A_HwAg1Meas/HwAg1Meas/HwAg1MeasPer3/Snsr1Read/RawHwAgRead/NewMsg/NoStsFlt ==
  note: Information Only:
      |
      | - Sensor Internal Fault (Status and Communication Nibble)
  Snsr1FCCN : Inport
  Snsr1Id : Inport  Port=2
  Snsr1Data : Inport  Port=3
  Action Port : ActionPort  ActionType=then
  Bus Creator : BusCreator  Inputs=3
  Bus Selector : BusSelector  OutputSignals=RawHwAg,TestOk,ParamByte
  Bus Selector1 : BusSelector  OutputSignals=RawHwAg,TestOk,ParamByte
  CommFlt : Subsystem  RequirementInfo={'linktype_rmi_doors' '0000cf44 (/ESG Group/FDD Module Requirements/EA4 Specific/CM670A_HwAg1Meas)' '#CM670A_28' 'true' 'REQ: CM670A_28' '' ; 'linktype_rmi_doors' '0000cf44 (/ESG Group/FDD Module Requirements/EA4 Specific/CM670A_HwAg1Meas)' '#CM670A_71' 'true' 'REQ: CM670A_71' '' } %GIDa_6d6f6192_7e1e_4a59_861e_4b877f73ea5a  TreatAsAtomicUnit=on
      mask Display: disp('CommFlt')
  CopyRight2 : Subsystem  Description=|  mask(Copyright Information){none=on}
      | Copyright info block.                                               
      |                                                                     
      | Place copyright information at the top of every subsystem in design.
      mask prompts: none "No parameters"
      mask help: Place copyright information at the top of every subsystem in design.
      mask Display:
      | NxtrConf = 'Nexteer Confidential';
      | 
      | sys = bdroot; %handle for the current model ("system")
      | first = get_param(sys,'Created');
      | first = first(end-3:end);  %year is last four digits
      | 
      | last = get_param(sys,'LastModifiedDate');
      | if isempty(last)
      |     last = datestr(now,'yyyy');
      | else
      |     last = last(end-3:end);
      | end
      | 
      | if strcmp(first,last)
      |     fprintf('%s -- Copyright %s Nexteer',NxtrConf,first)
      | else
      |     fprintf('%s -- %s%s- %s Nexteer',NxtrConf,char(169),first,last)
      | end
  If : If  IfExpression=u1 == 0
  Merge : Merge
  Merge1 : Merge
  Merge2 : Merge
  TestPass : Subsystem  TreatAsAtomicUnit=on
  Out1 : Outport
  wires:
  Snsr1FCCN/1 -> If/1
  If/1 -> TestPass/Action
  If/2 -> CommFlt/Action
  Merge/1 -> Bus Creator/2  "TestOk"
  Merge1/1 -> Bus Creator/3  "ParamByte"
  Merge2/1 -> Bus Creator/1  "RawHwAg"
  TestPass/1(Out1) -> Bus Selector/1
  CommFlt/1(Out2) -> Bus Selector1/1
  Bus Selector1/1 -> Merge2/1  "<RawHwAg>"
  Bus Selector/1 -> Merge2/2  "<RawHwAg>"
  Bus Selector1/2 -> Merge/1  "<TestOk>"
  Bus Selector1/3 -> Merge1/1  "<ParamByte>"
  Bus Selector/2 -> Merge/2  "<TestOk>"
  Bus Selector/3 -> Merge1/2  "<ParamByte>"
  Bus Creator/1 -> Out1/1
  Snsr1Data/1 -> TestPass/2(Snsr1Data)
  Snsr1Id/1 -> TestPass/1(Snsr1Id)

== system CM670A_HwAg1Meas/HwAg1Meas/HwAg1MeasPer3/Snsr1Read/RawHwAgRead/NewMsg/STSFLT ==
  Action Port : ActionPort  ActionType=else
  Add : Sum
  Bus Creator : BusCreator  Inputs=3
  Constant : Constant  OutDataTypeStr=uint8
  CopyRight2 : Subsystem  Description=|  mask(Copyright Information){none=on}
      | Copyright info block.                                               
      |                                                                     
      | Place copyright information at the top of every subsystem in design.
      mask prompts: none "No parameters"
      mask help: Place copyright information at the top of every subsystem in design.
      mask Display:
      | NxtrConf = 'Nexteer Confidential';
      | 
      | sys = bdroot; %handle for the current model ("system")
      | first = get_param(sys,'Created');
      | first = first(end-3:end);  %year is last four digits
      | 
      | last = get_param(sys,'LastModifiedDate');
      | if isempty(last)
      |     last = datestr(now,'yyyy');
      | else
      |     last = last(end-3:end);
      | end
      | 
      | if strcmp(first,last)
      |     fprintf('%s -- Copyright %s Nexteer',NxtrConf,first)
      | else
      |     fprintf('%s -- %s%s- %s Nexteer',NxtrConf,char(169),first,last)
      | end
  Data Store Read : DataStoreRead  DataStoreName=HwAg1Snsr1ComStsErrCntr
  Data Store Write : DataStoreWrite  DataStoreName=HwAg1Snsr1ComStsErrCntr
  Data Type Conversion : DataTypeConversion  OutDataTypeStr=uint8
  HwAg : Constant  Value=0  OutDataTypeStr=uint16
  NtcSts : simulink/Sources/Enumerated Constant  OutDataTypeStr=Enum: NtcSts1  Value=NtcSts1.NTCSTS_PREFAILD  SampleTime=inf
  PRTCL_FAULT : Constant  Value=ELECGLBPRM_PRTCLFLT_CNT_U08  OutDataTypeStr=uint8
  Signal Conversion : SignalConversion
  Out1 : Outport
  wires:
  PRTCL_FAULT/1 -> Bus Creator/3  "ParamByte"
  NtcSts/1 -> Data Type Conversion/1
  HwAg/1 -> Bus Creator/1  "RawHwAg"
  Bus Creator/1 -> Signal Conversion/1
  Signal Conversion/1 -> Out1/1
  Data Type Conversion/1 -> Bus Creator/2  "TestOk"
  Data Store Read/1 -> Add/1
  Constant/1 -> Add/2
  Add/1 -> Data Store Write/1

== system CM670A_HwAg1Meas/HwAg1Meas/HwAg1MeasPer3/Snsr1Read/RawHwAgRead/NoNewMsg/CopyRight2 ==

== system CM670A_HwAg1Meas/HwAg1Meas/HwAg1MeasPer3/Snsr1Read/SyncPulse/GetRefTmr1MicroSec32bit/CopyRight2 ==

== system CM670A_HwAg1Meas/HwAg1Meas/HwAg1MeasPer3/Snsr1Read/SyncPulse/GetTiSpan1MicroSec32bit/CopyRight2 ==

== system CM670A_HwAg1Meas/HwAg1Meas/HwAg1MeasPer4/HwAgRead/If Action Subsystem/AdjStepCalc/CopyRight2 ==

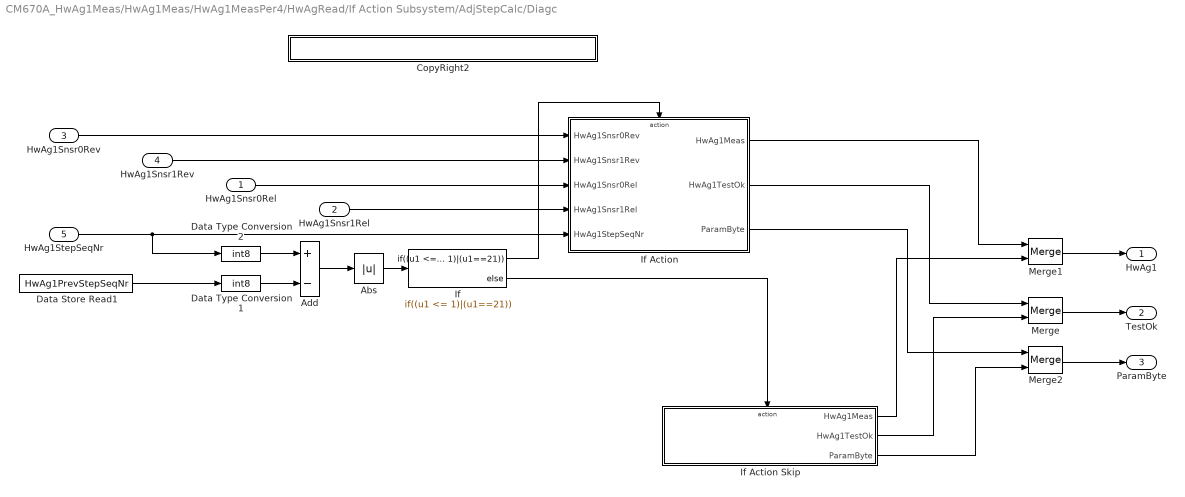
== system CM670A_HwAg1Meas/HwAg1Meas/HwAg1MeasPer4/HwAgRead/If Action Subsystem/AdjStepCalc/Diagc ==
  HwAg1Snsr0Rel : Inport
  HwAg1Snsr1Rel : Inport  Port=2
  HwAg1Snsr0Rev : Inport  Port=3
  HwAg1Snsr1Rev : Inport  Port=4
  HwAg1StepSeqNr : Inport  Port=5
  Abs : Abs
  Add : Sum  Inputs=+-
  CopyRight2 : Subsystem  Description=|  mask(Copyright Information){none=on}
      | Copyright info block.                                               
      |                                                                     
      | Place copyright information at the top of every subsystem in design.
      mask prompts: none "No parameters"
      mask help: Place copyright information at the top of every subsystem in design.
      mask Display:
      | NxtrConf = 'Nexteer Confidential';
      | 
      | sys = bdroot; %handle for the current model ("system")
      | first = get_param(sys,'Created');
      | first = first(end-3:end);  %year is last four digits
      | 
      | last = get_param(sys,'LastModifiedDate');
      | if isempty(last)
      |     last = datestr(now,'yyyy');
      | else
      |     last = last(end-3:end);
      | end
      | 
      | if strcmp(first,last)
      |     fprintf('%s -- Copyright %s Nexteer',NxtrConf,first)
      | else
      |     fprintf('%s -- %s%s- %s Nexteer',NxtrConf,char(169),first,last)
      | end
  Data Store Read1 : DataStoreRead  DataStoreName=HwAg1PrevStepSeqNr
  Data Type Conversion1 : DataTypeConversion  OutDataTypeStr=int8
  Data Type Conversion2 : DataTypeConversion  OutDataTypeStr=int8
  If : If  IfExpression=(u1 <= 1)|(u1==21)
  "If Action " : Subsystem  TreatAsAtomicUnit=on
  If Action Skip : Subsystem  RequirementInfo={'linktype_rmi_doors' '0000cf44 (/ESG Group/FDD Module Requirements/EA4 Specific/CM670A_HwAg1Meas)' '#CM670A_97' 'true' 'REQ: CM670A_97' '' } %GIDa_d763d448_3308_4803_9d41_af8d19d81401  TreatAsAtomicUnit=on
  Merge : Merge
  Merge1 : Merge
  Merge2 : Merge
  HwAg1 : Outport  OutDataTypeStr=single
  TestOk : Outport  Port=2  OutDataTypeStr=uint8
  ParamByte : Outport  Port=3  OutDataTypeStr=uint8
  wires:
  HwAg1StepSeqNr/1 -> Data Type Conversion2/1, "If Action "/5(HwAg1StepSeqNr)
  Add/1 -> Abs/1
  Abs/1 -> If/1
  If/1 -> "If Action "/Action
  If/2 -> If Action Skip/Action
  Merge/1 -> TestOk/1
  Merge2/1 -> ParamByte/1
  Merge1/1 -> HwAg1/1
  "If Action "/1(HwAg1Meas) -> Merge1/1
  If Action Skip/1(HwAg1Meas) -> Merge1/2
  "If Action "/2(HwAg1TestOk) -> Merge/1
  If Action Skip/2(HwAg1TestOk) -> Merge/2
  "If Action "/3(ParamByte) -> Merge2/1
  If Action Skip/3(ParamByte) -> Merge2/2
  Data Store Read1/1 -> Data Type Conversion1/1
  HwAg1Snsr0Rev/1 -> "If Action "/1(HwAg1Snsr0Rev)
  HwAg1Snsr1Rev/1 -> "If Action "/2(HwAg1Snsr1Rev)
  HwAg1Snsr0Rel/1 -> "If Action "/3(HwAg1Snsr0Rel)
  HwAg1Snsr1Rel/1 -> "If Action "/4(HwAg1Snsr1Rel)
  Data Type Conversion2/1 -> Add/1
  Data Type Conversion1/1 -> Add/2

== system CM670A_HwAg1Meas/HwAg1Meas/HwAg1MeasPer4/HwAgRead/If Action Subsystem/AdjStepCalc/InitStep ==
  HwAg1StepSeqNr_In : Inport
  CopyRight2 : Subsystem  Description=|  mask(Copyright Information){none=on}
      | Copyright info block.                                               
      |                                                                     
      | Place copyright information at the top of every subsystem in design.
      mask prompts: none "No parameters"
      mask help: Place copyright information at the top of every subsystem in design.
      mask Display:
      | NxtrConf = 'Nexteer Confidential';
      | 
      | sys = bdroot; %handle for the current model ("system")
      | first = get_param(sys,'Created');
      | first = first(end-3:end);  %year is last four digits
      | 
      | last = get_param(sys,'LastModifiedDate');
      | if isempty(last)
      |     last = datestr(now,'yyyy');
      | else
      |     last = last(end-3:end);
      | end
      | 
      | if strcmp(first,last)
      |     fprintf('%s -- Copyright %s Nexteer',NxtrConf,first)
      | else
      |     fprintf('%s -- %s%s- %s Nexteer',NxtrConf,char(169),first,last)
      | end
  Data Store Read1 : DataStoreRead  DataStoreName=HwAg1InitStepSeqNrCmpl
  DoNothing : Subsystem  TreatAsAtomicUnit=on
  Else : Subsystem  TreatAsAtomicUnit=on
  If : If  IfExpression=u1 == 0
  HwAg1StepSeqNr_Out : Outport
  wires:
  HwAg1StepSeqNr_In/1 -> HwAg1StepSeqNr_Out/1, Else/1(HwAg1StepSeqNr)
  Data Store Read1/1 -> If/1
  If/2 -> DoNothing/Action
  If/1 -> Else/Action

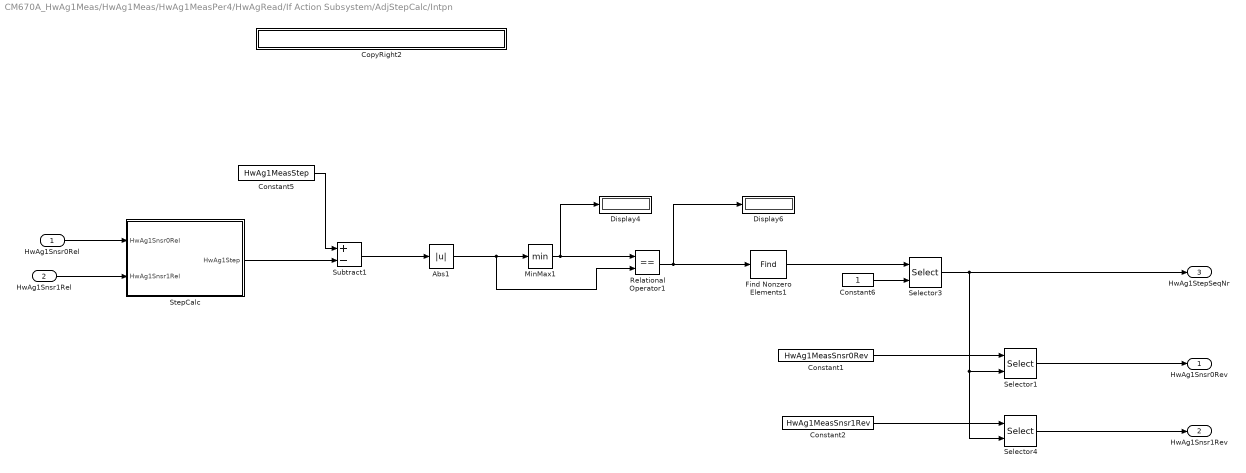
== system CM670A_HwAg1Meas/HwAg1Meas/HwAg1MeasPer4/HwAgRead/If Action Subsystem/AdjStepCalc/Intpn ==
  HwAg1Snsr0Rel : Inport
  HwAg1Snsr1Rel : Inport  Port=2
  Abs1 : Abs
  Constant1 : Constant  Value=HwAg1MeasSnsr0Rev  OutDataTypeStr=int16
  Constant2 : Constant  Value=HwAg1MeasSnsr1Rev  OutDataTypeStr=int16
  Constant5 : Constant  Value=HwAg1MeasStep  OutDataTypeStr=int16
  Constant6 : Constant
  CopyRight2 : Subsystem  Description=|  mask(Copyright Information){none=on}
      | Copyright info block.                                               
      |                                                                     
      | Place copyright information at the top of every subsystem in design.
      mask prompts: none "No parameters"
      mask help: Place copyright information at the top of every subsystem in design.
      mask Display:
      | NxtrConf = 'Nexteer Confidential';
      | 
      | sys = bdroot; %handle for the current model ("system")
      | first = get_param(sys,'Created');
      | first = first(end-3:end);  %year is last four digits
      | 
      | last = get_param(sys,'LastModifiedDate');
      | if isempty(last)
      |     last = datestr(now,'yyyy');
      | else
      |     last = last(end-3:end);
      | end
      | 
      | if strcmp(first,last)
      |     fprintf('%s -- Copyright %s Nexteer',NxtrConf,first)
      | else
      |     fprintf('%s -- %s%s- %s Nexteer',NxtrConf,char(169),first,last)
      | end
  Display4 : Display
  Display6 : Display
  Find Nonzero Elements1 : Find  NumberOfInputDimensions=4  OutDataTypeStr=uint8
  MinMax1 : MinMax
  Relational Operator1 : RelationalOperator  Operator===  OutDataTypeStr=boolean
  Selector1 : Selector  InputPortWidth=22  IndexOptions=Index vector (port)  Indices=[1 3]  OutputSizes=1
  Selector3 : Selector  InputPortWidth=22  IndexOptions=Index vector (port)  Indices=[1 3]  OutputSizes=1
  Selector4 : Selector  InputPortWidth=22  IndexOptions=Index vector (port)  Indices=[1 3]  OutputSizes=1
  StepCalc : Subsystem
  Subtract1 : Sum  Inputs=+-
  HwAg1Snsr0Rev : Outport
  HwAg1Snsr1Rev : Outport  Port=2
  HwAg1StepSeqNr : Outport  Port=3
  wires:
  Selector3/1 -> HwAg1StepSeqNr/1, Selector4/2, Selector1/2
  Subtract1/1 -> Abs1/1
  Constant5/1 -> Subtract1/1
  Abs1/1 -> Relational Operator1/2, MinMax1/1
  Find Nonzero Elements1/1 -> Selector3/1
  Relational Operator1/1 -> Display6/1, Find Nonzero Elements1/1
  MinMax1/1 -> Relational Operator1/1, Display4/1
  Constant6/1 -> Selector3/2
  Constant1/1 -> Selector1/1
  Constant2/1 -> Selector4/1
  Selector1/1 -> HwAg1Snsr0Rev/1
  Selector4/1 -> HwAg1Snsr1Rev/1
  StepCalc/1(HwAg1Step) -> Subtract1/2
  HwAg1Snsr0Rel/1 -> StepCalc/1(HwAg1Snsr0Rel)
  HwAg1Snsr1Rel/1 -> StepCalc/2(HwAg1Snsr1Rel)

== system CM670A_HwAg1Meas/HwAg1Meas/HwAg1MeasPer4/HwAgRead/If Action Subsystem/DebStepSelection/CopyRight2 ==

== system CM670A_HwAg1Meas/HwAg1Meas/HwAg1MeasPer4/HwAgRead/If Action Subsystem/HwAg1Snsr0RelCalc/CopyRight2 ==

== system CM670A_HwAg1Meas/HwAg1Meas/HwAg1MeasPer4/HwAgRead/If Action Subsystem/HwAg1Snsr1RelCalc/CopyRight2 ==

== system CM670A_HwAg1Meas/HwAg1Meas/HwAg1MeasPer4/HwAgRead/If Action Subsystem/SetNtcSts/CopyRight2 ==
